simulink model "IQImbalanceFilter3tap"  (R2013a)
settings: Solver=ode45  StartTime=0.0  StopTime=10.0  RelTol=1e-3
settings Model: Creator=USER  LastModifiedBy=USER

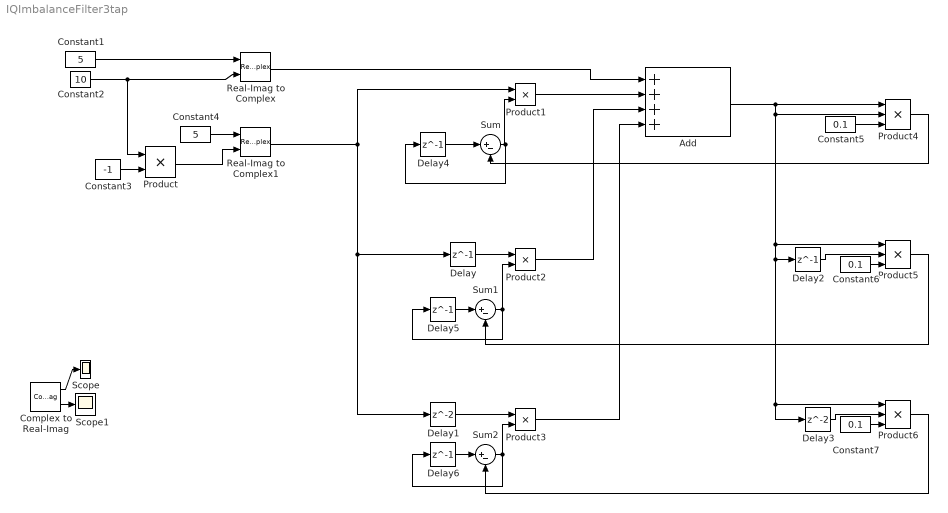
== system IQImbalanceFilter3tap ==
  Add : Sum  Inputs=++++
  Complex to Real-Imag : ComplexToRealImag
  Constant1 : Constant  Value=5
  Constant2 : Constant  Value=10
  Constant3 : Constant  Value=-1
  Constant4 : Constant  Value=5
  Constant5 : Constant  Value=0.1
  Constant6 : Constant  Value=0.1
  Constant7 : Constant  Value=0.1
  Delay{,2,4..6} (5 alike) : Delay  DelayLength=1
  Delay1 : Delay
  Delay3 : Delay
  Product{,1..3} (4 alike) : Product  SampleTime=1
  Product4 : Product  Inputs=3  SampleTime=1
  Product5 : Product  Inputs=3  SampleTime=1
  Product6 : Product  Inputs=3  SampleTime=1
  Real-Imag to Complex : RealImagToComplex  SampleTime=1
  Real-Imag to Complex1 : RealImagToComplex  SampleTime=1
  Scope : Scope
  Scope1 : Scope
  Sum : Sum  Inputs=|+-
  Sum1 : Sum  Inputs=|+-
  Sum2 : Sum  Inputs=|+-
  wires:
  Constant2/1 -> Product/1, Real-Imag to Complex/2
  Constant3/1 -> Product/2
  Product/1 -> Real-Imag to Complex1/2
  Constant1/1 -> Real-Imag to Complex/1
  Constant4/1 -> Real-Imag to Complex1/1
  Complex to Real-Imag/1 -> Scope/1
  Complex to Real-Imag/2 -> Scope1/1
  Real-Imag to Complex/1 -> Add/1
  Real-Imag to Complex1/1 -> Delay1/1, Delay/1, Product1/1
  Delay1/1 -> Product3/1
  Product1/1 -> Add/2
  Product2/1 -> Add/3
  Product3/1 -> Add/4
  Add/1 -> Delay2/1, Delay3/1, Product6/1, Product5/1, Product4/2, Product4/1
  Delay2/1 -> Product5/2
  Delay3/1 -> Product6/2
  Product4/1 -> Sum/2
  Sum/1 -> Delay4/1, Product1/2
  Delay4/1 -> Sum/1
  Delay/1 -> Product2/1
  Product5/1 -> Sum1/2
  Sum1/1 -> Product2/2, Delay5/1
  Delay5/1 -> Sum1/1
  Delay6/1 -> Sum2/1
  Product6/1 -> Sum2/2
  Sum2/1 -> Delay6/1, Product3/2
  Constant5/1 -> Product4/3
  Constant6/1 -> Product5/3
  Constant7/1 -> Product6/3
